simulink model "mpc_simscape222"  (R2018b)
settings: Solver=ode45  StartTime=0.0  StopTime=1  RelTol=1e-3
libraries: nesl_utility x17, fl_lib x13, pe_lib x10, elec_lib x9, powerlib_meascontrol x4, simulink x1, pePwmGenerator x1, powerlib x1
settings Model: Creator=zero  LastModifiedBy=zero

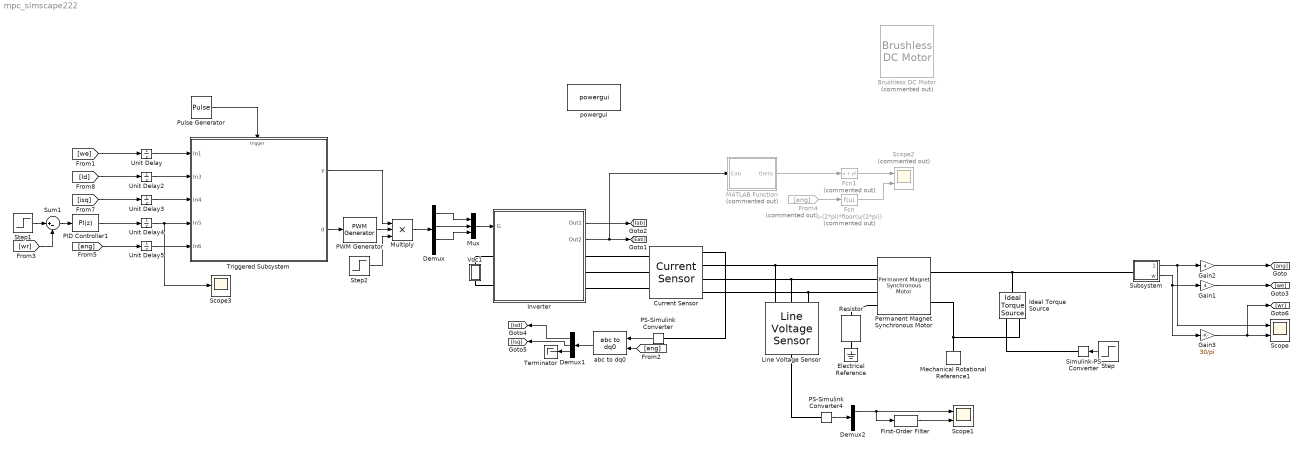
== system mpc_simscape222 ==
  Brushless DC Motor : pe_lib/Machines/Permanent Magnet Rotor/Brushless DC Motor  Commented=on  rotor_param=1  pm_flux_linkage=0.00689 Wb  theta_constant=pi/8 rad  emf_max=9.6 V  DphiDtheta_tab=[0, -.1528, -.1528, .1528, .1528, 0] Wb/rad  back_emf_tab=[0, -9.6, -9.6, 9.6, 9.6, 0] V  rotor_angle_tab=[0, 7.5, 22.5, 37.5, 52.5, 60] deg  w_meas=600 rpm  nPolePairs=4  stator_param=1  Ld=0.0002 H  Lq=0.0002 H  L0=0.00016 H  Ls=0.0002 H  Lm=0 H  Ms=0.00002 H  Rs=0.375 Ohm  zero_sequence=pe.enum.park.zerosequence.exclude  J=2e-6 kg*m^2  lam=1e-6 N*m/(rad/s)  axes_param=1  i_d_specify=off  i_d_priority=None  i_d=0 A  i_d_nominal_specify=off  i_d_nominal_unit=A  i_d_nominal_value=1  i_q_specify=off  i_q_priority=None  i_q=0 A  i_q_nominal_specify=off  i_q_nominal_unit=A  i_q_nominal_value=1  torque_specify=off  torque_priority=None  torque=0 N*m  torque_nominal_specify=off  torque_nominal_unit=N*m  torque_nominal_value=1  angular_velocity_specify=off  angular_velocity_priority=High  angular_velocity=0 rpm  angular_velocity_nominal_specify=off  angular_velocity_nominal_unit=rpm  angular_velocity_nominal_value=1  angular_position_specify=off  angular_position_priority=High  angular_position=0 deg  angular_position_nominal_specify=off  angular_position_nominal_unit=deg  angular_position_nominal_value=1
      settings: SourceProductName=Simscape Power Systems  SourceProductBaseCode=PS
  Current Sensor : pe_lib/Sensors/Current Sensor
      settings: SourceProductName=Simscape Power Systems  SourceProductBaseCode=PS
  Demux : Demux  Outputs=6
  Demux1 : Demux  Outputs=3
  Demux2 : Demux  Outputs=3
  Electrical Reference : fl_lib/Electrical/Electrical Elements/Electrical Reference
  Fcn : Fcn  Commented=on  Expr=u-(2*pi)*floor(u/(2*pi))
  Fcn1 : Fcn  Commented=on  Expr=u + pi
  First-Order Filter : powerlib_meascontrol/Filters/First-Order Filter  FilterType=Lowpass  Tc=1e-3  Ts=0  Initialize=off  Vac_Init=[0, 0, 60]  Vdc_Init=0  PlotResponse=off  FreqRange="[0,  200,  1]"
      settings: SourceProductName=Simscape Power Systems
  From4 : From  Commented=on  GotoTag=ang
  Gain1 : Gain  Gain=4
  Gain2 : Gain  Gain=4
  Gain3 : Gain  Gain=30/pi
  Ideal Torque Source : fl_lib/Mechanical/Mechanical Sources/Ideal Torque Source
  Inverter : Subsystem
  Line Voltage Sensor : pe_lib/Sensors/Line Voltage Sensor
      settings: SourceProductName=Simscape Power Systems  SourceProductBaseCode=PS
  MATLAB Function : MATLAB Function  Commented=on  TreatAsAtomicUnit=on
  Mechanical Rotational Reference1 : fl_lib/Mechanical/Rotational Elements/Mechanical Rotational Reference
  Multiply : Product  Inputs=3
  Mux : Mux  Inputs=3
  PID Controller1 : simulink/Continuous/PID Controller  Controller=PI  Form=Parallel  TimeDomain=Discrete-time  SampleTime=0.08e-3  IntegratorMethod=Forward Euler  FilterMethod=Forward Euler  ControllerParametersSource=internal  P=0.005  I=0.12  D=5  UseFilter=on  N=100  TunerSelectOption=Transfer Function Based (PID Tuner App)  InitialConditionSource=internal  InitialConditionForIntegrator=0  InitialConditionForFilter=0  DifferentiatorICPrevScaledInput=0  ExternalReset=none  TrackingMode=off  Kt=1  LimitOutput=off  UpperSaturationLimit=0.5  LowerSaturationLimit=-0.5  LinearizeAsGain=on  AntiWindupMode=clamping  Kb=1  POutMin=[]  POutMax=[]  IOutMin=[]  IOutMax=[]  DOutMin=[]  DOutMax=[]  NOutMin=[]  NOutMax=[]  SumOutMin=[]  SumOutMax=[]  SaturationOutMin=[]  SaturationOutMax=[]  PParamMin=[]  PParamMax=[]  IParamMin=[]  IParamMax=[]  DParamMin=[]  DParamMax=[]  NParamMin=[]  NParamMax=[]  KbParamMin=[]  KbParamMax=[]  KtParamMin=[]  KtParamMax=[]  KbOutMin=[]  KbOutMax=[]  KtOutMin=[]  KtOutMax=[]  IntegratorOutMin=[]  IntegratorOutMax=[]  FilterOutMin=[]  FilterOutMax=[]  SumI1OutMin=[]  SumI1OutMax=[]  SumI2OutMin=[]  SumI2OutMax=[]  SumI3OutMin=[]  SumI3OutMax=[]  SumI4OutMin=[]  SumI4OutMax=[]  SumDOutMin=[]  SumDOutMax=[]  DifferentiatorOutMin=[]  DifferentiatorOutMax=[]  FilterDiffOutCoefMin=[]  FilterDiffOutCoefMax=[]  ReciprocalOutMin=[]  ReciprocalOutMax=[]  SumDenOutMin=[]  SumDenOutMax=[]  SumNumOutMin=[]  SumNumOutMax=[]  DivideOutMin=[]  DivideOutMax=[]  IntegratorContinuousStateAttributes=''  IntegratorStateMustResolveToSignalObject=off  IntegratorRTWStateStorageClass=Auto  FilterContinuousStateAttributes=''  FilterStateMustResolveToSignalObject=off  FilterRTWStateStorageClass=Auto  ParallelPVariant=InternalParameters  IdealPVariant=Disabled  IVariant=InternalParameters  DVariant=Disabled  IntegratorVariant=Discrete  SatVariant=Disabled  AWVariant=Passthrough  PCopyVariant=Disabled  TRVariant=Disabled  FdbkBlocksVariant=Forward  IdealPFdbkVariant=Disabled  SatFdbkVariant=Disabled  DerivativeFilterVariant=Disabled  NVariant=Disabled  NCopyVariant=Disabled_SignalSpec  FilterICVariant=Disabled  IntegratorICVariant=InternalICs  ExternalResetVariant=Disabled  TRSumVariant=Passthrough  SumFdbkVariant=Disabled  SumVariant=Sum_PI
  PS-Simulink Converter : nesl_utility/PS-Simulink Converter  PhysicalDomain=network_engine_domain  SubClassName=ps_output  LeftPortType=input  RightPortType=output  PseudoPeriodic=off  Frequencies=[]  Unit=1  AffineConversion=off
  PS-Simulink Converter4 : nesl_utility/PS-Simulink Converter  PhysicalDomain=network_engine_domain  SubClassName=ps_output  LeftPortType=input  RightPortType=output  PseudoPeriodic=off  Frequencies=[]  Unit=1  AffineConversion=off
  PWM Generator : pePwmGenerator/PWM Generator  CarrCount=Up  Tper=1/20000  Ts=1/200000
  Permanent Magnet Synchronous Motor : pe_lib/Machines/Permanent Magnet Rotor/Permanent Magnet Synchronous Motor  nPolePairs=4  pmflux_param=1  pm_flux_linkage=0.0068916 Wb  torque_constant=0.04 N*m/A  back_emf_constant=0.0041 V/rpm  stator_param=1  Ld=0.2 mH  Lq=0.2 mH  L0=0 H  Ls=0.0002 H  Lm=-0.00002 H  Ms=0.00002 H  Rs=0.375 Ohm  zero_sequence=pe.enum.park.zerosequence.exclude  J=2.6e-6 kg*m^2  lam=1.3e-6 N*m/(rad/s)  axes_param=pe.enum.rotorangle.qaxis  i_d_specify=off  i_d_priority=None  i_d=0 A  i_d_nominal_specify=off  i_d_nominal_unit=A  i_d_nominal_value=1  i_q_specify=off  i_q_priority=None  i_q=0 A  i_q_nominal_specify=off  i_q_nominal_unit=A  i_q_nominal_value=1  torque_specify=off  torque_priority=None  torque=0 N*m  torque_nominal_specify=off  torque_nominal_unit=N*m  torque_nominal_value=1  angular_velocity_specify=off  angular_velocity_priority=High  angular_velocity=0 rpm  angular_velocity_nominal_specify=off  angular_velocity_nominal_unit=rpm  angular_velocity_nominal_value=1  angular_position_specify=off  angular_position_priority=High  angular_position=0 deg  angular_position_nominal_specify=off  angular_position_nominal_unit=deg  angular_position_nominal_value=1
      settings: SourceProductName=Simscape Power Systems  SourceProductBaseCode=PS
  Pulse Generator : DiscretePulseGenerator  PulseType=Time based  Period=80e-6  PulseWidth=5
  Resistor : elec_lib/Passive Devices/Resistor  R=10 kOhm  R_tol=5  enable_R_tol=0  tol_distribution=1  nSigma=4  enable_operating_limits=0  operating_limit_action=2  max_working_voltage=100 V  power_rating=1 W  enable_faults=0  fault_action=1  R_faulted=inf Ohm  enable_temporal_fault=0  t_fault=1 s  enable_behavioral_fault=0  max_permissible_current=1 A  t_fail_on_current=1 s  noise_mode=0  sample_time=1e-3 s  repeatability=1  auto_seed=3873088395  user_seed=0  Tdevice=25 degC  alpha=3.93e-3 1/K  Tmeas=25 degC  thermal_mass=100 J/K  power_derating_T1=70 degC  power_derating_T2=155 degC  operating_temperature_range_vec=[-50, 150] degC  temperature_specify=off  temperature_priority=High  temperature=298.15 K  temperature_nominal_specify=off  temperature_nominal_unit=K  temperature_nominal_value=1
  Scope : Scope  NumInputPorts=2
  Scope1 : Scope  NumInputPorts=2
  Scope2 : Scope  Commented=on  NumInputPorts=2
  Scope3 : Scope
  Simulink-PS Converter : nesl_utility/Simulink-PS Converter  PhysicalDomain=network_engine_domain  SubClassName=ps_input  LeftPortType=input  RightPortType=output  PseudoPeriodic=off  Frequencies=[]  NoiseDistribution=none  NoiseParameters=[]  Unit=1  AffineConversion=off  FilteringAndDerivatives=provide  SimscapeFilterOrder=1  InputFilterTimeConstant=0.001  UdotUserProvided=0
  Step : Step  Time=0.1  After=-0.01  SampleTime=0
  Step1 : Step  Time=0.025  After=1600  SampleTime=0
  Step2 : Step  Time=0.1  Before=1  SampleTime=0
  Subsystem : Subsystem
  Sum1 : Sum  Inputs=|+-
  Terminator : Terminator
  Triggered Subsystem : Subsystem  TreatAsAtomicUnit=on
  Unit Delay{,2..5} (5 alike) : UnitDelay  SampleTime=-1
  Vdc1 : Subsystem
  abc to dq0 : powerlib_meascontrol/Transformations/abc to dq0  Alignment=90 degrees behind phase A axis
  powergui : powerlib/powergui  Priority=1  SimulationMode=Discrete  SampleTime=3e-7  frequency=60  Iterations=50  frequencyindice=60  Pbase=100e6  ErrMax=1e-4  UnitsV=kV  UnitsW=MW  buscounter=0  FunctionMessages=off  echomessages=off  EnableUseOfTLC=off  CurrentSourceSwitches=off  DisableSnubberDevices=off  DisableRonSwitches=off  DisableVfSwitches=off  DisplayEquations=off  SolverType=Tustin/Backward Euler (TBE)  Interpol=off  ExternalGateDelay=off  methode=off  Ts=100  x0status=blocks  SPID=on  SwTol=0  HookPort=off  RestoreLinks=warning  ResistiveCurrentMeasurement=off  Frange=[0:2:500]  Ylog=off  Xlog=on  ShowGrid=off  save=off  variable=ZData  structure=0  ZoomFFT=off  StartTime=0.0  cycles=1  DisplayStyle=1  fundamental=60  FreqAxis=off  MaxFrequency=1000  frequencyindicesteady=1  RmsSteady=1  display=off
  wires:
  Inverter/2(Out2) -> MATLAB Function/1(Eab), [Eab]
  Inverter/1(Out1) -> [Iab]
  Subsystem/1(theta) -> Gain2/1, Scope/1
  Mux/1 -> Inverter/1(G)
  Triggered Subsystem/2(d) -> PWM Generator/1
  PWM Generator/1 -> Multiply/2
  Multiply/1 -> Demux/1
  Demux/1 -> Mux/1
  Demux/3 -> Mux/2
  Demux/5 -> Mux/3
  [ang] -> abc to dq0/2
  Demux1/3 -> Terminator/1
  Pulse Generator/1 -> Triggered Subsystem/Trigger
  Unit Delay5/1 -> Triggered Subsystem/5(In6)
  Unit Delay2/1 -> Triggered Subsystem/2(In3)
  [we] -> Unit Delay/1
  [Id] -> Unit Delay2/1
  [ang] -> Unit Delay5/1
  Step1/1 -> Sum1/1
  Sum1/1 -> PID Controller1/1
  [isq] -> Unit Delay3/1
  Unit Delay3/1 -> Triggered Subsystem/3(In4)
  Unit Delay/1 -> Triggered Subsystem/1(In1)
  Triggered Subsystem/1(y) -> Multiply/1
  [wr] -> Sum1/2
  Gain1/1 -> [we]
  Subsystem/2(w) -> Gain3/1, Gain1/1
  Gain3/1 -> [wr], Scope/2
  Step/1 -> Simulink-PS Converter/1
  PID Controller1/1 -> Unit Delay4/1
  MATLAB Function/1(theta) -> Fcn1/1
  From4/1 -> Fcn/1
  Fcn/1 -> Scope2/2
  Fcn1/1 -> Scope2/1
  Unit Delay4/1 -> Scope3/1, Triggered Subsystem/4(In5)
  Step2/1 -> Multiply/3
  PS-Simulink Converter/1 -> abc to dq0/1
  Gain2/1 -> [ang]
  PS-Simulink Converter4/1 -> Demux2/1
  Demux2/1 -> First-Order Filter/1, Scope1/1
  First-Order Filter/1 -> Scope1/2
  Demux1/1 -> [isd]
  Demux1/2 -> [isq]
  abc to dq0/1 -> Demux1/1
  connections:
  Line Voltage Sensor/LConn1 -- Permanent Magnet Synchronous Motor/LConn1 -- Current Sensor/RConn2
  Line Voltage Sensor/LConn2 -- Permanent Magnet Synchronous Motor/LConn2 -- Current Sensor/RConn3
  Line Voltage Sensor/LConn3 -- Permanent Magnet Synchronous Motor/LConn3 -- Current Sensor/RConn4
  Electrical Reference/LConn1 -- Resistor/RConn1
  Vdc1/LConn1 -- Inverter/LConn1
  Permanent Magnet Synchronous Motor/LConn4 -- Resistor/LConn1
  Mechanical Rotational Reference1/LConn1 -- Permanent Magnet Synchronous Motor/RConn2 -- Ideal Torque Source/RConn2
  PS-Simulink Converter4/LConn1 -- Line Voltage Sensor/RConn1
  Ideal Torque Source/LConn1 -- Permanent Magnet Synchronous Motor/RConn1 -- Subsystem/LConn1
  Inverter/LConn2 -- Vdc1/RConn1
  Current Sensor/LConn1 -- Inverter/RConn1
  Current Sensor/LConn2 -- Inverter/RConn2
  Current Sensor/LConn3 -- Inverter/RConn3
  PS-Simulink Converter/LConn1 -- Current Sensor/RConn1
  Simulink-PS Converter/RConn1 -- Ideal Torque Source/RConn1

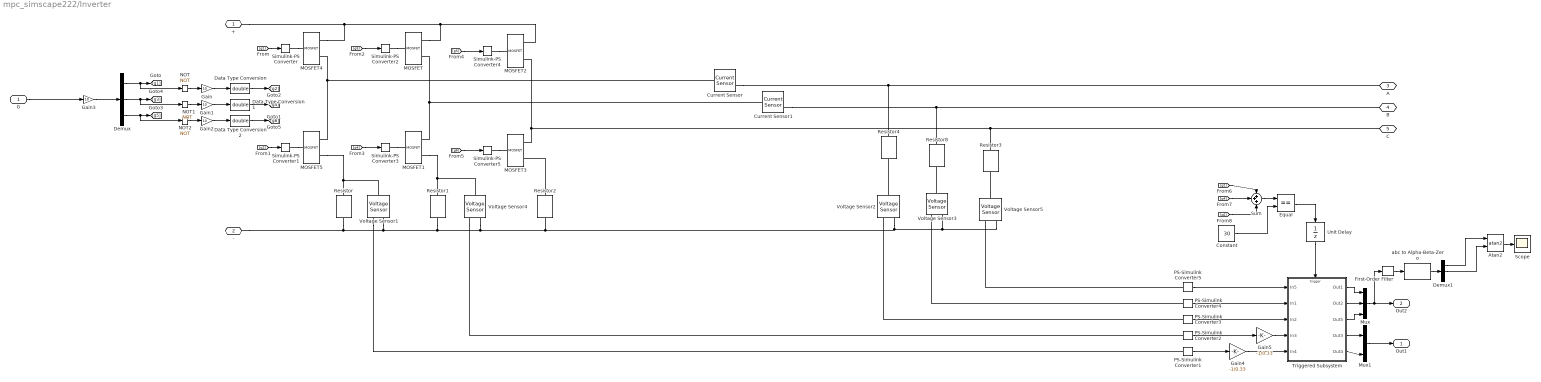
== system mpc_simscape222/Inverter ==
  G : Inport
  Atan2 : Trigonometry  Operator=atan2
  Constant : Constant  Value=30
  Current Sensor : fl_lib/Electrical/Electrical Sensors/Current Sensor
  Current Sensor1 : fl_lib/Electrical/Electrical Sensors/Current Sensor
  Data Type Conversion : DataTypeConversion  OutDataTypeStr=double
  Data Type Conversion1 : DataTypeConversion  OutDataTypeStr=double
  Data Type Conversion2 : DataTypeConversion  OutDataTypeStr=double
  Demux : Demux  Outputs=3
  Demux1 : Demux  Outputs=3
  Equal : RelationalOperator  Operator===  OutDataTypeStr=boolean  RndMeth=Simplest
  First-Order Filter : powerlib_meascontrol/Filters/First-Order Filter  FilterType=Lowpass  Tc=10e-3  Ts=0  Initialize=on  Vac_Init=[0, 0, 60]  Vdc_Init=0  PlotResponse=off  FreqRange="[0,  200,  1]"
      settings: SourceProductName=Simscape Power Systems
  Gain{,1..3} (4 alike) : Gain  Gain=10
  Gain4 : Gain  Gain=-1/0.33
  Gain5 : Gain  Gain=-1/0.33
  MOSFET : pe_lib/Semiconductors/Fundamental Components/MOSFET  Rds=0.01 Ohm  Goff=1e-6 1/Ohm  Vth=2 V  diode_param=2  diode_Vf=0.8 V  diode_Ron=0.001 Ohm  diode_Goff=1e-5 1/Ohm  diode_C=5e-8 F  diode_iRM=-235 A  diode_iF=300 A  diode_idot=-50 A/us  diode_trr_param=1  diode_trr_factor=3  diode_trr=15 us  diode_Qrr=1.5e+3 s*uA  thermal_loss_option=2  Voff=300 V  Tau=1e-4 s  Tj=[ 298.15 398.15 ] K  Iout_scalar=600 A  Eon_scalar=0.02286 J  Eoff_scalar=0.01714 J  Von_scalar=2.7 V  Iout_data=[ 0 10 50 100 200 400 600 ] A  Eon_data=[ 0 2.9e-4 0.00143 0.00286 0.00571 0.01314 0.02286; 0 5.7e-4 0.00263 0.00514 0.01029 0.02057 0.03029 ] J  Eoff_data=[ 0 2.1e-4 0.00107 0.00214 0.00429 0.009859999999999999 0.01714; 0 4.3e-4 0.00197 0.00386 0.00771 0.01543 0.02271 ] J  Von_data=[ 0 1.1 1.3 1.45 1.75 2.25 2.7; 0 1 1.15 1.35 1.7 2.35 3 ] V
      settings: SourceProductName=Simscape Power Systems  SourceProductBaseCode=PS
  MOSFET1 : pe_lib/Semiconductors/Fundamental Components/MOSFET  Rds=0.01 Ohm  Goff=1e-6 1/Ohm  Vth=2 V  diode_param=2  diode_Vf=0.8 V  diode_Ron=0.001 Ohm  diode_Goff=1e-5 1/Ohm  diode_C=5e-8 F  diode_iRM=-235 A  diode_iF=300 A  diode_idot=-50 A/us  diode_trr_param=1  diode_trr_factor=3  diode_trr=15 us  diode_Qrr=1.5e+3 s*uA  thermal_loss_option=2  Voff=300 V  Tau=1e-4 s  Tj=[ 298.15 398.15 ] K  Iout_scalar=600 A  Eon_scalar=0.02286 J  Eoff_scalar=0.01714 J  Von_scalar=2.7 V  Iout_data=[ 0 10 50 100 200 400 600 ] A  Eon_data=[ 0 2.9e-4 0.00143 0.00286 0.00571 0.01314 0.02286; 0 5.7e-4 0.00263 0.00514 0.01029 0.02057 0.03029 ] J  Eoff_data=[ 0 2.1e-4 0.00107 0.00214 0.00429 0.009859999999999999 0.01714; 0 4.3e-4 0.00197 0.00386 0.00771 0.01543 0.02271 ] J  Von_data=[ 0 1.1 1.3 1.45 1.75 2.25 2.7; 0 1 1.15 1.35 1.7 2.35 3 ] V
      settings: SourceProductName=Simscape Power Systems  SourceProductBaseCode=PS
  MOSFET{2..5} (4 alike) : pe_lib/Semiconductors/Fundamental Components/MOSFET  Rds=0.0003 Ohm  Goff=1e-6 1/Ohm  Vth=2 V  diode_param=2  diode_Vf=0.8 V  diode_Ron=0.001 Ohm  diode_Goff=1e-5 1/Ohm  diode_C=5e-8 F  diode_iRM=-235 A  diode_iF=300 A  diode_idot=-50 A/us  diode_trr_param=1  diode_trr_factor=3  diode_trr=15 us  diode_Qrr=1.5e+3 s*uA  thermal_loss_option=2  Voff=300 V  Tau=1e-4 s  Tj=[ 298.15 398.15 ] K  Iout_scalar=600 A  Eon_scalar=0.02286 J  Eoff_scalar=0.01714 J  Von_scalar=2.7 V  Iout_data=[ 0 10 50 100 200 400 600 ] A  Eon_data=[ 0 2.9e-4 0.00143 0.00286 0.00571 0.01314 0.02286; 0 5.7e-4 0.00263 0.00514 0.01029 0.02057 0.03029 ] J  Eoff_data=[ 0 2.1e-4 0.00107 0.00214 0.00429 0.009859999999999999 0.01714; 0 4.3e-4 0.00197 0.00386 0.00771 0.01543 0.02271 ] J  Von_data=[ 0 1.1 1.3 1.45 1.75 2.25 2.7; 0 1 1.15 1.35 1.7 2.35 3 ] V
      settings: SourceProductName=Simscape Power Systems  SourceProductBaseCode=PS
  Mux : Mux  Inputs=3
  Mux1 : Mux  Inputs=2
  NOT : Logic  Operator=NOT  IconShape=distinctive  AllPortsSameDT=off  OutDataTypeStr=boolean
  NOT1 : Logic  Operator=NOT  IconShape=distinctive  AllPortsSameDT=off  OutDataTypeStr=boolean
  NOT2 : Logic  Operator=NOT  IconShape=distinctive  AllPortsSameDT=off  OutDataTypeStr=boolean
  PS-Simulink Converter{1..5} (5 alike) : nesl_utility/PS-Simulink Converter  PhysicalDomain=network_engine_domain  SubClassName=ps_output  LeftPortType=input  RightPortType=output  PseudoPeriodic=off  Frequencies=[]  Unit=1  AffineConversion=off
  Resistor : elec_lib/Passive Devices/Resistor  R=0.33 Ohm  R_tol=5  enable_R_tol=0  tol_distribution=1  nSigma=4  enable_operating_limits=0  operating_limit_action=2  max_working_voltage=100 V  power_rating=1 W  enable_faults=0  fault_action=1  R_faulted=inf Ohm  enable_temporal_fault=0  t_fault=1 s  enable_behavioral_fault=0  max_permissible_current=1 A  t_fail_on_current=1 s  noise_mode=0  sample_time=1e-3 s  repeatability=1  auto_seed=1983148915  user_seed=0  Tdevice=25 degC  alpha=3.93e-3 1/K  Tmeas=25 degC  thermal_mass=100 J/K  power_derating_T1=70 degC  power_derating_T2=155 degC  operating_temperature_range_vec=[-50, 150] degC  temperature_specify=off  temperature_priority=High  temperature=298.15 K  temperature_nominal_specify=off  temperature_nominal_unit=K  temperature_nominal_value=1
  Resistor1 : elec_lib/Passive Devices/Resistor  R=0.33 Ohm  R_tol=5  enable_R_tol=0  tol_distribution=1  nSigma=4  enable_operating_limits=0  operating_limit_action=2  max_working_voltage=100 V  power_rating=1 W  enable_faults=0  fault_action=1  R_faulted=inf Ohm  enable_temporal_fault=0  t_fault=1 s  enable_behavioral_fault=0  max_permissible_current=1 A  t_fail_on_current=1 s  noise_mode=0  sample_time=1e-3 s  repeatability=1  auto_seed=130519863  user_seed=0  Tdevice=25 degC  alpha=3.93e-3 1/K  Tmeas=25 degC  thermal_mass=100 J/K  power_derating_T1=70 degC  power_derating_T2=155 degC  operating_temperature_range_vec=[-50, 150] degC  temperature_specify=off  temperature_priority=High  temperature=298.15 K  temperature_nominal_specify=off  temperature_nominal_unit=K  temperature_nominal_value=1
  Resistor2 : elec_lib/Passive Devices/Resistor  R=0.33 Ohm  R_tol=5  enable_R_tol=0  tol_distribution=1  nSigma=4  enable_operating_limits=0  operating_limit_action=2  max_working_voltage=100 V  power_rating=1 W  enable_faults=0  fault_action=1  R_faulted=inf Ohm  enable_temporal_fault=0  t_fault=1 s  enable_behavioral_fault=0  max_permissible_current=1 A  t_fail_on_current=1 s  noise_mode=0  sample_time=1e-3 s  repeatability=1  auto_seed=3006660371  user_seed=0  Tdevice=25 degC  alpha=3.93e-3 1/K  Tmeas=25 degC  thermal_mass=100 J/K  power_derating_T1=70 degC  power_derating_T2=155 degC  operating_temperature_range_vec=[-50, 150] degC  temperature_specify=off  temperature_priority=High  temperature=298.15 K  temperature_nominal_specify=off  temperature_nominal_unit=K  temperature_nominal_value=1
  Resistor3 : elec_lib/Passive Devices/Resistor  R=10 kOhm  R_tol=5  enable_R_tol=0  tol_distribution=1  nSigma=4  enable_operating_limits=0  operating_limit_action=2  max_working_voltage=100 V  power_rating=1 W  enable_faults=0  fault_action=1  R_faulted=inf Ohm  enable_temporal_fault=0  t_fault=1 s  enable_behavioral_fault=0  max_permissible_current=1 A  t_fail_on_current=1 s  noise_mode=0  sample_time=1e-3 s  repeatability=1  auto_seed=3568381785  user_seed=0  Tdevice=25 degC  alpha=3.93e-3 1/K  Tmeas=25 degC  thermal_mass=100 J/K  power_derating_T1=70 degC  power_derating_T2=155 degC  operating_temperature_range_vec=[-50, 150] degC  temperature_specify=off  temperature_priority=High  temperature=298.15 K  temperature_nominal_specify=off  temperature_nominal_unit=K  temperature_nominal_value=1
  Resistor4 : elec_lib/Passive Devices/Resistor  R=10 kOhm  R_tol=5  enable_R_tol=0  tol_distribution=1  nSigma=4  enable_operating_limits=0  operating_limit_action=2  max_working_voltage=100 V  power_rating=1 W  enable_faults=0  fault_action=1  R_faulted=inf Ohm  enable_temporal_fault=0  t_fault=1 s  enable_behavioral_fault=0  max_permissible_current=1 A  t_fail_on_current=1 s  noise_mode=0  sample_time=1e-3 s  repeatability=1  auto_seed=921323082  user_seed=0  Tdevice=25 degC  alpha=3.93e-3 1/K  Tmeas=25 degC  thermal_mass=100 J/K  power_derating_T1=70 degC  power_derating_T2=155 degC  operating_temperature_range_vec=[-50, 150] degC  temperature_specify=off  temperature_priority=High  temperature=298.15 K  temperature_nominal_specify=off  temperature_nominal_unit=K  temperature_nominal_value=1
  Resistor8 : elec_lib/Passive Devices/Resistor  R=10 kOhm  R_tol=5  enable_R_tol=0  tol_distribution=1  nSigma=4  enable_operating_limits=0  operating_limit_action=2  max_working_voltage=100 V  power_rating=1 W  enable_faults=0  fault_action=1  R_faulted=inf Ohm  enable_temporal_fault=0  t_fault=1 s  enable_behavioral_fault=0  max_permissible_current=1 A  t_fail_on_current=1 s  noise_mode=0  sample_time=1e-3 s  repeatability=1  auto_seed=3653638066  user_seed=0  Tdevice=25 degC  alpha=3.93e-3 1/K  Tmeas=25 degC  thermal_mass=100 J/K  power_derating_T1=70 degC  power_derating_T2=155 degC  operating_temperature_range_vec=[-50, 150] degC  temperature_specify=off  temperature_priority=High  temperature=298.15 K  temperature_nominal_specify=off  temperature_nominal_unit=K  temperature_nominal_value=1
  Scope : Scope
  Simulink-PS Converter{,1..5} (6 alike) : nesl_utility/Simulink-PS Converter  PhysicalDomain=network_engine_domain  SubClassName=ps_input  LeftPortType=input  RightPortType=output  PseudoPeriodic=off  Frequencies=[]  NoiseDistribution=none  NoiseParameters=[]  Unit=1  AffineConversion=off  FilteringAndDerivatives=provide  SimscapeFilterOrder=1  InputFilterTimeConstant=0.001  UdotUserProvided=0
  Sum : Sum  Inputs=+++
  Triggered Subsystem : Subsystem  TreatAsAtomicUnit=on
  Unit Delay : UnitDelay  SampleTime=1/400000
  Voltage Sensor{1..5} (5 alike) : fl_lib/Electrical/Electrical Sensors/Voltage Sensor
  abc to Alpha-Beta-Zero : powerlib_meascontrol/Transformations/abc to Alpha-Beta-Zero
      settings: SourceProductName=Simscape Power Systems
  + : PMIOPort  Side=Left
  - : PMIOPort  Port=2  Side=Left
  A : PMIOPort  Port=3  Side=Right
  B : PMIOPort  Port=4  Side=Right
  C : PMIOPort  Port=5  Side=Right
  Out1 : Outport
  Out2 : Outport  Port=2
  wires:
  G/1 -> Gain3/1
  [g1] -> Simulink-PS Converter/1
  [g2] -> Simulink-PS Converter1/1
  [g3] -> Simulink-PS Converter2/1
  [g4] -> Simulink-PS Converter3/1
  [g5] -> Simulink-PS Converter4/1
  [g6] -> Simulink-PS Converter5/1
  Demux/1 -> NOT/1, [g1]
  Demux/2 -> NOT1/1, [g3]
  Demux/3 -> NOT2/1, [g5]
  NOT/1 -> Gain/1
  NOT1/1 -> Gain1/1
  NOT2/1 -> Gain2/1
  Gain/1 -> Data Type Conversion/1
  Gain1/1 -> Data Type Conversion1/1
  Gain2/1 -> Data Type Conversion2/1
  Data Type Conversion/1 -> [g2]
  Data Type Conversion1/1 -> [g4]
  Data Type Conversion2/1 -> [g6]
  PS-Simulink Converter3/1 -> Triggered Subsystem/3(In2)
  Gain3/1 -> Demux/1
  PS-Simulink Converter1/1 -> Gain4/1
  PS-Simulink Converter2/1 -> Gain5/1
  Triggered Subsystem/2(Out2) -> Mux/2
  Triggered Subsystem/1(Out1) -> Mux/1
  Triggered Subsystem/4(Out3) -> Mux1/1
  Triggered Subsystem/5(Out4) -> Mux1/2
  PS-Simulink Converter4/1 -> Triggered Subsystem/2(In1)
  Gain4/1 -> Triggered Subsystem/5(In4)
  Gain5/1 -> Triggered Subsystem/4(In3)
  [g2] -> Sum/1
  [g6] -> Sum/3
  [g4] -> Sum/2
  Sum/1 -> Equal/1
  Constant/1 -> Equal/2
  Equal/1 -> Unit Delay/1
  Mux/1 -> First-Order Filter/1, Out2/1
  Mux1/1 -> Out1/1
  Unit Delay/1 -> Triggered Subsystem/Trigger
  PS-Simulink Converter5/1 -> Triggered Subsystem/1(In5)
  Triggered Subsystem/3(Out5) -> Mux/3
  Atan2/1 -> Scope/1
  abc to Alpha-Beta-Zero/1 -> Demux1/1
  Demux1/1 -> Atan2/1
  Demux1/2 -> Atan2/2
  First-Order Filter/1 -> abc to Alpha-Beta-Zero/1
  connections:
  Current Sensor/RConn2 -- Resistor4/LConn1 -- A/RConn1
  MOSFET/RConn1 -- MOSFET2/RConn1 -- MOSFET4/RConn1 -- +/RConn1
  MOSFET3/RConn1 -- C/RConn1 -- Resistor3/LConn1 -- MOSFET2/RConn2
  Current Sensor1/RConn2 -- B/RConn1 -- Resistor8/LConn1
  Simulink-PS Converter/RConn1 -- MOSFET4/LConn1
  Simulink-PS Converter1/RConn1 -- MOSFET5/LConn1
  Simulink-PS Converter2/RConn1 -- MOSFET/LConn1
  Simulink-PS Converter3/RConn1 -- MOSFET1/LConn1
  Simulink-PS Converter4/RConn1 -- MOSFET2/LConn1
  Simulink-PS Converter5/RConn1 -- MOSFET3/LConn1
  MOSFET5/RConn2 -- Voltage Sensor1/LConn1 -- Resistor/LConn1
  MOSFET1/RConn2 -- Voltage Sensor4/LConn1 -- Resistor1/LConn1
  PS-Simulink Converter3/LConn1 -- Voltage Sensor2/RConn1
  PS-Simulink Converter4/LConn1 -- Voltage Sensor3/RConn1
  Resistor2/LConn1 -- MOSFET3/RConn2
  MOSFET5/RConn1 -- Current Sensor/LConn1 -- MOSFET4/RConn2
  MOSFET1/RConn1 -- Current Sensor1/LConn1 -- MOSFET/RConn2
  Voltage Sensor3/LConn1 -- Resistor8/RConn1
  Voltage Sensor2/LConn1 -- Resistor4/RConn1
  PS-Simulink Converter2/LConn1 -- Voltage Sensor4/RConn1
  Voltage Sensor1/RConn1 -- PS-Simulink Converter1/LConn1
  Voltage Sensor5/LConn1 -- Resistor3/RConn1
  Voltage Sensor5/RConn2 -- Voltage Sensor2/RConn2 -- -/RConn1 -- Resistor/RConn1 -- Voltage Sensor1/RConn2 -- Resistor1/RConn1 -- Voltage Sensor4/RConn2 -- Resistor2/RConn1 -- Voltage Sensor3/RConn2
  PS-Simulink Converter5/LConn1 -- Voltage Sensor5/RConn1

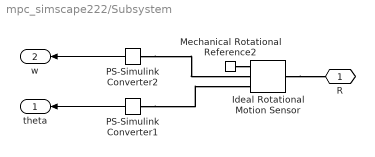
== system mpc_simscape222/Subsystem ==
  Ideal Rotational Motion Sensor : fl_lib/Mechanical/Mechanical Sensors/Ideal Rotational Motion Sensor  offset=0 rad
  Mechanical Rotational Reference2 : fl_lib/Mechanical/Rotational Elements/Mechanical Rotational Reference
  PS-Simulink Converter1 : nesl_utility/PS-Simulink Converter  PhysicalDomain=network_engine_domain  SubClassName=ps_output  LeftPortType=input  RightPortType=output  PseudoPeriodic=off  Frequencies=[]  Unit=1  AffineConversion=off
  PS-Simulink Converter2 : nesl_utility/PS-Simulink Converter  PhysicalDomain=network_engine_domain  SubClassName=ps_output  LeftPortType=input  RightPortType=output  PseudoPeriodic=off  Frequencies=[]  Unit=1  AffineConversion=off
  R : PMIOPort  Side=Left
  theta : Outport
  w : Outport  Port=2
  wires:
  PS-Simulink Converter1/1 -> theta/1
  PS-Simulink Converter2/1 -> w/1
  connections:
  Ideal Rotational Motion Sensor/LConn1 -- R/RConn1
  Mechanical Rotational Reference2/LConn1 -- Ideal Rotational Motion Sensor/RConn1
  PS-Simulink Converter2/LConn1 -- Ideal Rotational Motion Sensor/RConn2
  PS-Simulink Converter1/LConn1 -- Ideal Rotational Motion Sensor/RConn3

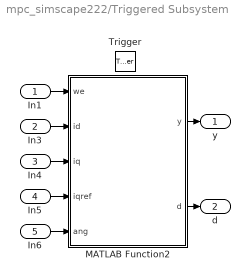
== system mpc_simscape222/Triggered Subsystem ==
  In1 : Inport
  In3 : Inport  Port=2
  In4 : Inport  Port=3
  In5 : Inport  Port=4
  In6 : Inport  Port=5
  Trigger : TriggerPort  VariantControl=Variant
  MATLAB Function2 : MATLAB Function  TreatAsAtomicUnit=on
  y : Outport
  d : Outport  Port=2
  wires:
  MATLAB Function2/1(y) -> y/1
  In1/1 -> MATLAB Function2/1(we)
  In3/1 -> MATLAB Function2/2(id)
  In4/1 -> MATLAB Function2/3(iq)
  In5/1 -> MATLAB Function2/4(iqref)
  In6/1 -> MATLAB Function2/5(ang)
  MATLAB Function2/2(d) -> d/1

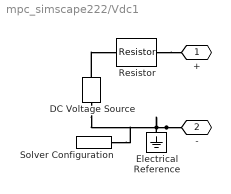
== system mpc_simscape222/Vdc1 ==
  DC Voltage Source : elec_lib/Additional Components/SPICE-Compatible Components/Sources/DC Voltage Source  DC=12 V
      settings: SourceProductName=Simscape Electronics  SourceProductBaseCode=SN
  Electrical Reference : fl_lib/Electrical/Electrical Elements/Electrical Reference
  Resistor : elec_lib/Passive Devices/Resistor  R=0.001 Ohm  R_tol=5  enable_R_tol=0  tol_distribution=1  nSigma=4  enable_operating_limits=0  operating_limit_action=2  max_working_voltage=100 V  power_rating=1 W  enable_faults=0  fault_action=1  R_faulted=inf Ohm  enable_temporal_fault=0  t_fault=1 s  enable_behavioral_fault=0  max_permissible_current=1 A  t_fail_on_current=1 s  noise_mode=0  sample_time=1e-3 s  repeatability=1  auto_seed=1801814819  user_seed=0  Tdevice=25 degC  alpha=3.93e-3 1/K  Tmeas=25 degC  thermal_mass=100 J/K  power_derating_T1=70 degC  power_derating_T2=155 degC  operating_temperature_range_vec=[-50, 150] degC  temperature_specify=off  temperature_priority=High  temperature=298.15 K  temperature_nominal_specify=off  temperature_nominal_unit=K  temperature_nominal_value=1
  Solver Configuration : nesl_utility/Solver Configuration  PhysicalDomain=network_engine_domain  SubClassName=solver  LeftPortType=input  RightPortType=generic  Tones=[]  Harmonics=[]  SimulateNoise=off  Profile=off  UseLocalSampling=off  EnableSwitchedLinearOptims=on  FrequencyDomain=off  UseCCode=off  RelTol=0.001  AbsTol=1e-06  MinStep=1e-09  ToWorkspace=off  RevertToSquareIcSolve=off  NumHomotopyIterations=100  PhasorMode=off  PhasorModeNumHarmonics=1  DoDC=off  ResidualTolerance=1e-09  UseLocalSolver=off  LocalSolverChoice=NE_BACKWARD_EULER_ADVANCER  LocalSolverSampleTime=0.001  DoFixedCost=off  MaxNonlinIter=3  MaxModeIter=2  LinearAlgebra=auto  EquationFormulation=NE_TIME_EF  DelaysMemoryBudget=1024  AutomaticFiltering=on  FilteringTimeConstant=0.001  PartitionStorageMethod=AS_NEEDED  PartitionMemoryBudget=1024
  + : PMIOPort  Side=Left
  - : PMIOPort  Port=2  Side=Right
  connections:
  Resistor/RConn1 -- +/RConn1
  -/RConn1 -- Electrical Reference/LConn1 -- DC Voltage Source/RConn1 -- Solver Configuration/RConn1
  DC Voltage Source/LConn1 -- Resistor/LConn1

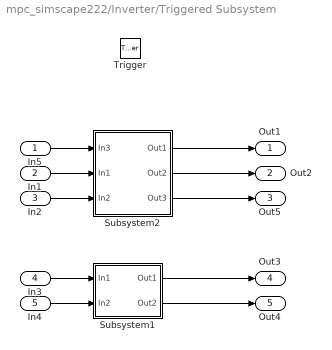
== system mpc_simscape222/Inverter/Triggered Subsystem ==
  In5 : Inport
  In1 : Inport  Port=2
  In2 : Inport  Port=3
  In3 : Inport  Port=4
  In4 : Inport  Port=5
  Trigger : TriggerPort  VariantControl=Variant
  Subsystem1 : Subsystem
  Subsystem2 : Subsystem
  Out1 : Outport
  Out2 : Outport  Port=2
  Out5 : Outport  Port=3
  Out3 : Outport  Port=4
  Out4 : Outport  Port=5
  wires:
  Subsystem2/1(Out1) -> Out1/1
  In1/1 -> Subsystem2/2(In1)
  In2/1 -> Subsystem2/3(In2)
  Subsystem2/2(Out2) -> Out2/1
  Subsystem1/2(Out2) -> Out4/1
  In4/1 -> Subsystem1/2(In2)
  In3/1 -> Subsystem1/1(In1)
  Subsystem1/1(Out1) -> Out3/1
  In5/1 -> Subsystem2/1(In3)
  Subsystem2/3(Out3) -> Out5/1

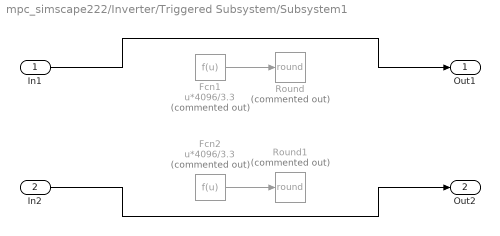
== system mpc_simscape222/Inverter/Triggered Subsystem/Subsystem1 ==
  In1 : Inport
  In2 : Inport  Port=2
  Fcn1 : Fcn  Commented=on  Expr=u*4096/3.3
  Fcn2 : Fcn  Commented=on  Expr=u*4096/3.3
  Round : Rounding  Commented=on  Operator=round
  Round1 : Rounding  Commented=on  Operator=round
  Out1 : Outport
  Out2 : Outport  Port=2
  wires:
  In1/1 -> Out1/1
  Fcn2/1 -> Round1/1
  Fcn1/1 -> Round/1
  In2/1 -> Out2/1

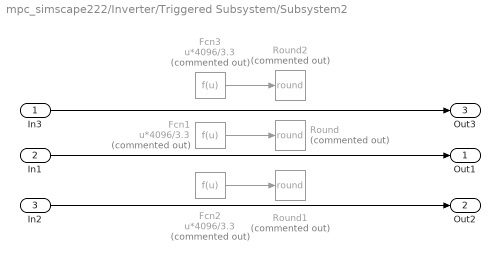
== system mpc_simscape222/Inverter/Triggered Subsystem/Subsystem2 ==
  In3 : Inport
  In1 : Inport  Port=2
  In2 : Inport  Port=3
  Fcn1 : Fcn  Commented=on  Expr=u*4096/3.3
  Fcn2 : Fcn  Commented=on  Expr=u*4096/3.3
  Fcn3 : Fcn  Commented=on  Expr=u*4096/3.3
  Round : Rounding  Commented=on  Operator=round
  Round1 : Rounding  Commented=on  Operator=round
  Round2 : Rounding  Commented=on  Operator=round
  Out1 : Outport
  Out2 : Outport  Port=2
  Out3 : Outport  Port=3
  wires:
  In2/1 -> Out2/1
  Fcn1/1 -> Round/1
  Fcn2/1 -> Round1/1
  In1/1 -> Out1/1
  In3/1 -> Out3/1
  Fcn3/1 -> Round2/1

== matlab function mpc_simscape222/Triggered Subsystem/MATLAB Function2 ==
  data: y output; we input; id input; iq input; iqref input; ang input; d output
function [y,d]  = MPC(we,id,iq,iqref,ang)

persistent oldState;

if isempty(oldState)
    oldState = 1;
end

Ts = 80e-6;
Vdc = 12;
L = 0.0002;
R = 0.375;
psiPM = 0.0068916;

p = 0.7;
q = 0.4;
r = 0.6;
s = 0.8;

states =[1 0     0 1     0 1;
         1 0     1 0     0 1;
         0 1     1 0     0 1;
         0 1     1 0     1 0;
         0 1     0 1     1 0;
         1 0     0 1     1 0;];
%          p 0     0 p     0 p;
%          p 0     p 0     0 p;
%          0 p     p 0     0 p;
%          0 p     p 0     p 0;
%          0 p     0 p     p 0;
%          p 0     0 p     p 0;
%          q 0     0 q     0 q;
%          q 0     q 0     0 q;
%          0 q     q 0     0 q;
%          0 q     q 0     q 0;
%          0 q     0 q     q 0;
%          q 0     0 q     q 0;
%          r 0     0 r     0 r;
%          r 0     r 0     0 r;
%          0 r     r 0     0 r;
%          0 r     r 0     r 0;
%          0 r     0 r     r 0;
%          r 0     0 r     r 0;
%          s 0     0 s     0 s;
%          s 0     s 0     0 s;
%          0 s     s 0     0 s;
%          0 s     s 0     s 0;
%          0 s     0 s     s 0;
%          s 0     0 s     s 0;];

y = states(1,:)';
cost = [];

% id = (2/3)*[sin(ang) sin(ang - (2*pi/3)) sin(ang + (2*pi/3))]*[Iab(1) Iab(2) -(Iab(1)+Iab(2))]';
% iq = (2/3)*[cos(ang) cos(ang - (2*pi/3)) cos(ang + (2*pi/3))]*[Iab(1) Iab(2) -(Iab(1)+Iab(2))]';

for i=1:length(states)
    vsd = (2*Vdc/3)*[sin(ang) sin(ang - (2*pi/3)) sin(ang + (2*pi/3))]*states(i,[1,3,5])';
    vsq = (2*Vdc/3)*[cos(ang) cos(ang - (2*pi/3)) cos(ang + (2*pi/3))]*states(i,[1,3,5])';
    
    id_p = id;
    iq_p = iq;
    
    for x = 1:12
        id_p = ((1-(R*Ts/L))*id_p)+(Ts*we*iq_p)+(vsd*Ts/L);
        iq_p = ((1-(R*Ts/L))*iq_p)-(Ts*we*id_p)-(psiPM*we*Ts)+(vsq*Ts/L);
    end
    
    cost = [cost (id_p)^2 + (iqref - iq_p)^2];
end

a = find(cost == min(cost));
a = a(1);

d = max(states(a,:))*0.99;

oldState = a;
y = [states(a,:)>0]'*1;

== matlab function mpc_simscape222/MATLAB Function ==
  data: Eab input; theta output
function theta = fcn(Eab)
    a = Eab(1);
    b = Eab(2);
    c = -(a+b);
    Ealpha = (a*2/3) - ((b+c)/3);
	Ebeta = (b-c)*250/433;
    
    theta = atan2(Ebeta,Ealpha);
